simulink model "Commande_et_Modele"  (R2016b)
settings: Solver=ode5  StartTime=0.0  StopTime=inf  FixedStep=dt  RelTol=1e-3  EnableMultiTasking=on
values from neighbouring files (symbols this model uses):
  D = R/(i*C)*1000    (= 0.0129166666667)    [param.m]
  dt = 1e-4    (= 0.0001)    [param.m]
  Vsat = 10    [param.m]
undefined symbols (not defined in the file or in its folder): National_Instruments, PCIe
libraries: sldrtlib x4
settings Model: SimulationMode=external  ExtModeTrigDuration=100000  Creator=Fred  LastModifiedBy=Xavier
settings DataIOCC: LimitDataPoints=on  MaxDataPoints=10000  SaveFormat=Array  SignalLoggingSaveFormat=ModelDataLogs
settings OptimizationCC: ExpressionDepthLimit=2147483647
settings DebuggingCC: UnderspecifiedInitializationDetection=Classic  MergeDetectMultiDrivingBlocksExec=none  SolverPrmCheckMsg=warning  FcnCallInpInsideContextMsg=warning  StateNameClashWarn=warning  SFUnexpectedBacktrackingDiag=warning  SFNoUnconditionalDefaultTransitionDiag=warning  SFExecutionAtInitializationDiag=none
settings HardwareCC: TargetBitPerLong=64  TargetBitPerPointer=64  TargetIntDivRoundTo=Zero  TargetEndianess=LittleEndian  TargetWordSize=64  TargetHWDeviceType=Intel->x86-64
settings ModelReferenceCC: PropagateSignalLabelsOutOfModel=off
settings RTWCC: SystemTargetFile=sldrt.tlc  TemplateMakefile=sldrt.tmf  Description=Simulink Desktop Real-Time  RTWCompilerOptimization=on
settings CodeAppCC: MaxIdLength=95
settings SimulinkDesktopRealTimeCC: TargetPreCompLibLocation=C:\Program Files\MATLAB\R2016b\toolbox\sldrt\lib\win64  TargetLangStandard=C89/C90 (ANSI)  SupportVariableSizeSignals=off
settings ConfigComp: CovMetricSettings=dw  CovHtmlReporting=on  CovSaveCumulativeToWorkspaceVar=on  CovSaveSingleToWorkspaceVar=on  CovExternalEMLEnable=off  CovSFcnEnable=off

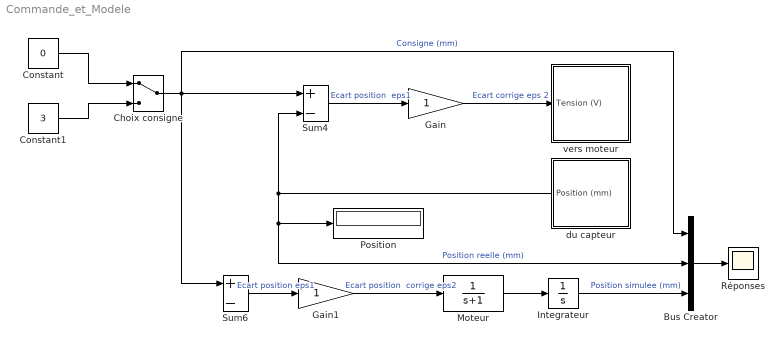
== system Commande_et_Modele ==
  Bus Creator : BusCreator  Inputs=3
  Choix consigne : ManualSwitch
  Constant : Constant  Value=0
  Constant1 : Constant  Value=3
  Gain : Gain
  Gain1 : Gain
  Integrateur : Integrator
  Moteur : TransferFcn  Denominator=[1 1]
  Position : Display
  Réponses : Scope
  Sum4 : Sum  Inputs=+-
  Sum6 : Sum  Inputs=+-
  du capteur : Subsystem
      mask Display: image(imread('carte.jpg'))
  vers moteur : Subsystem
      mask Display: image(imread('carte.jpg'))
  wires:
  du capteur/1(Position (mm)) -> Sum4/2, Position/1, Bus Creator/2  "Position reelle (mm)"
  Constant/1 -> Choix consigne/1
  Choix consigne/1 -> Sum6/1, Sum4/1, Bus Creator/1  "Consigne (mm)"
  Integrateur/1 -> Bus Creator/3  "Position simulee (mm)"
  Sum6/1 -> Gain1/1  "Ecart position eps1"
  Bus Creator/1 -> Réponses/1
  Constant1/1 -> Choix consigne/2
  Moteur/1 -> Integrateur/1
  Sum4/1 -> Gain/1  "Ecart position  eps1"
  Gain/1 -> vers moteur/1(Tension (V))  "Ecart corrige eps 2"
  Gain1/1 -> Moteur/1  "Ecart position  corrige eps2"

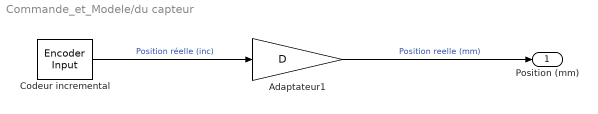
== system Commande_et_Modele/du capteur ==
  Adaptateur1 : Gain  Gain=D
  Codeur incremental : sldrtlib/Encoder Input  SampleTime=dt  MaxMissedTicks=10  ShowMissedTicks=off  YieldWhenWaiting=off  DrvName=National_Instruments/PCIe-6321  DrvAddress=4294967295  DrvOptions=[0 0 0 2 2 2 0]  Channels=1  QuadMode=3  IndexPulse=2  InputFilter=Inf  DataType=1
      settings: AttributesFormatString=National Instruments\nPCIe-6321 [auto]
  Position (mm) : Outport
  wires:
  Codeur incremental/1 -> Adaptateur1/1  "Position réelle (inc)"
  Adaptateur1/1 -> Position (mm)/1  "Position reelle (mm)"

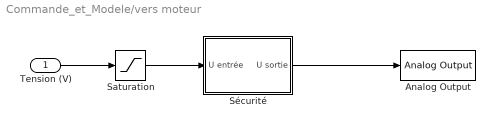
== system Commande_et_Modele/vers moteur ==
  Tension (V) : Inport
  Analog Output : sldrtlib/Analog Output  SampleTime=dt  MaxMissedTicks=10  ShowMissedTicks=off  YieldWhenWaiting=off  DrvName=National_Instruments/PCIe-6321  DrvAddress=4294967295  DrvOptions=[0 0 0 2 2 2 0]  Channels=1  RangeMode=1  VoltRange=1  InitialValue=[]  FinalValue=0
      settings: AttributesFormatString=National Instruments\nPCIe-6321 [auto]
  Saturation : Saturate  UpperLimit=10  LowerLimit=-10
  Sécurité : Subsystem
  wires:
  Sécurité/1(U sortie) -> Analog Output/1
  Saturation/1 -> Sécurité/1(U entrée)
  Tension (V)/1 -> Saturation/1

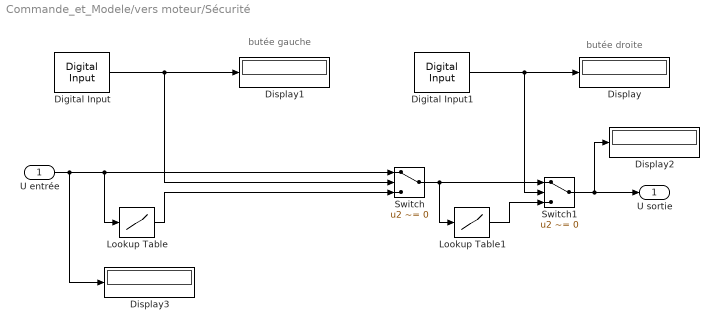
== system Commande_et_Modele/vers moteur/Sécurité ==
  note: butée gauche
  note: butée droite
  U entrée : Inport
  Digital Input : sldrtlib/Digital Input  SampleTime=dt  MaxMissedTicks=10  ShowMissedTicks=off  YieldWhenWaiting=off  DrvName=National_Instruments/PCIe-6321  DrvAddress=4294967295  DrvOptions=[0 0 0 2 2 2 0]  Channels=3  BitMode=1  DataType=9
      settings: AttributesFormatString=National Instruments\nPCIe-6321 [auto]
  Digital Input1 : sldrtlib/Digital Input  SampleTime=dt  MaxMissedTicks=10  ShowMissedTicks=off  YieldWhenWaiting=off  DrvName=National_Instruments/PCIe-6321  DrvAddress=4294967295  DrvOptions=[0 0 0 2 2 2 0]  Channels=2  BitMode=1  DataType=9
      settings: AttributesFormatString=National Instruments\nPCIe-6321 [auto]
  Display{,1..3} (4 alike) : Display
      Display settings: Decimation=3
      Display2 settings: Decimation=3
      Display3 settings: Decimation=3
  Lookup Table : Lookup  InputValues=[-Vsat 0 Vsat]  Table=[0 0 Vsat]
  Lookup Table1 : Lookup  InputValues=[-Vsat 0 Vsat]  Table=[-Vsat 0 0]
  Switch : Switch  Criteria=u2 ~= 0
  Switch1 : Switch  Criteria=u2 ~= 0
  U sortie : Outport
  wires:
  U entrée/1 -> Lookup Table/1, Switch/1, Display3/1
  Digital Input/1 -> Switch/2, Display1/1
  Lookup Table/1 -> Switch/3
  Switch/1 -> Switch1/1, Lookup Table1/1
  Digital Input1/1 -> Switch1/2, Display/1
  Lookup Table1/1 -> Switch1/3
  Switch1/1 -> U sortie/1, Display2/1
